simulink model "PH1_2converters_psv"  (R2017a)
settings: Solver=VariableStepAuto  StartTime=0.0  StopTime=.2  MaxStep=1e-4  RelTol=1e-3
libraries: powerlib x35, powerlib_meascontrol x2
settings Model: Creator=erich  LastModifiedBy=erich

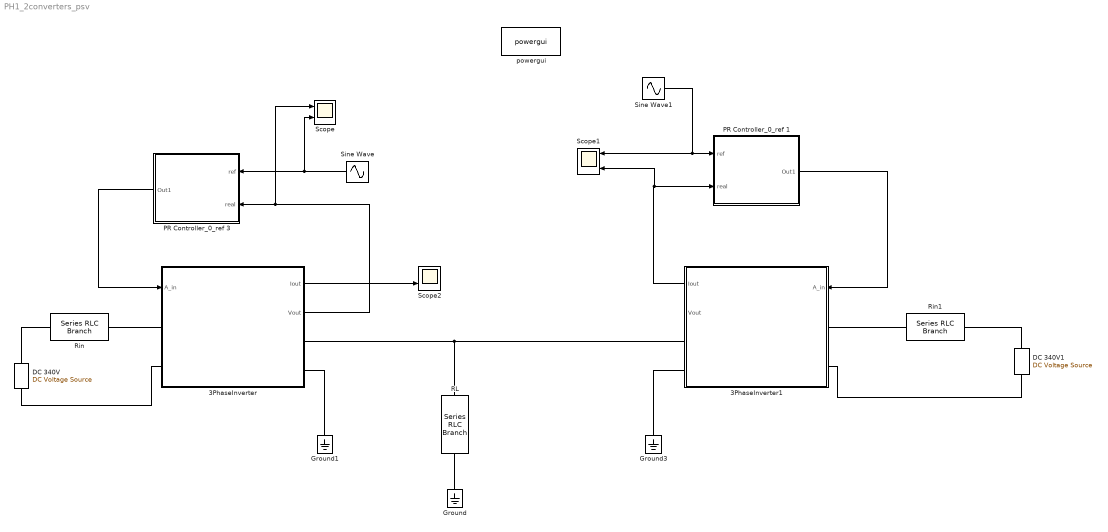
== system PH1_2converters_psv ==
  3PhaseInverter : Subsystem  mask{st_time=2e-3, f_sw=5000}
      mask prompts: st_time "Tiempo muerto (Start)"; f_sw "Switching frequency"
      mask Display:
      | port_label('input', 1, 'd', 'texmode', 'on')
      | 
      | port_label('lconn', 1, 'DC +')
      | port_label('lconn', 2, 'DC -')
      | 
      | 
      | port_label('rconn', 1, 'V_{out+}')
      | port_label('rconn', 2, 'B_{out-}')
      | 
      | 
      | port_label('output', 1, 'I_{out}', 'texmode', 'on')
      | port_label('output', 2, 'V_{out}', 'texmode', 'on')
      | 
      | plot([0.1 .9], [0.1 .9])
      | plot([0.2 .4], [.7 .7])
      | plot([0.2 .24], [.65 .65])
      | plot([0.28 .32], [.65 .65])
      | plot([0.36 .40], [.65 .65])
      | 
      | plot([.5:.01:.7], .25+sin(30*[.2:.01:.4])/10)
  3PhaseInverter1 : Subsystem  mask{st_time=.1, f_sw=5000}
      mask prompts: st_time "Tiempo muerto (Start)"; f_sw "Switching frequency"
      mask Display:
      | port_label('input', 1, 'd', 'texmode', 'on')
      | 
      | port_label('lconn', 1, 'DC +')
      | port_label('lconn', 2, 'DC -')
      | 
      | 
      | port_label('rconn', 1, 'V_{out+}')
      | port_label('rconn', 2, 'B_{out-}')
      | 
      | 
      | port_label('output', 1, 'I_{out}', 'texmode', 'on')
      | port_label('output', 2, 'V_{out}', 'texmode', 'on')
      | 
      | plot([0.1 .9], [0.1 .9])
      | plot([0.2 .4], [.7 .7])
      | plot([0.2 .24], [.65 .65])
      | plot([0.28 .32], [.65 .65])
      | plot([0.36 .40], [.65 .65])
      | 
      | plot([.5:.01:.7], .25+sin(30*[.2:.01:.4])/10)
  DC 340V : powerlib/Electrical Sources/DC Voltage Source  Amplitude=340  Measurements=None
  DC 340V1 : powerlib/Electrical Sources/DC Voltage Source  Amplitude=340  Measurements=None
  Ground : powerlib/Elements/Ground  LConnTagsString=a
  Ground1 : powerlib/Elements/Ground  LConnTagsString=a
  Ground3 : powerlib/Elements/Ground  LConnTagsString=a
  PR Controller_0_ref 1 : Subsystem  mask{Kp=1/100, Ki=7, wa=10, w0=60*2*pi, st_time=.1}
      mask prompts: Kp "Ganancia Proporcional"; Ki "Ganancia Integral"; wa "Ancho camapana resonancia"; w0 "Frecuencia Central"; st_time "Tiempo muerto (Start)"
      mask Display:
      | port_label('input',1,'ref')
      | port_label('input',2,'sens')
      | port_label('output',1,'out')
      | 
      | plot(.4+[0:.01:pi/10], .32+sin(40*[0:.01:pi/10])/13)
      | 
      | plot([.4 .6],.05+[.5 .7])
      | plot([.4 .6],.05+[.9 .7])
      | plot([.4 .4],.05+[.9 .5])
      | 
      | text(.27,.37,'\fontsize{25} \int', 'texmode', 'on')
  PR Controller_0_ref 3 : Subsystem  mask{Kp=1/100, Ki=1, wa=1, w0=60*2*pi, st_time=2e-3}
      mask prompts: Kp "Ganancia Proporcional"; Ki "Ganancia Integral"; wa "Ancho camapana resonancia"; w0 "Frecuencia Central"; st_time "Tiempo muerto (Start)"
      mask Display:
      | port_label('input',1,'ref')
      | port_label('input',2,'sens')
      | port_label('output',1,'out')
      | 
      | plot(.4+[0:.01:pi/10], .32+sin(40*[0:.01:pi/10])/13)
      | 
      | plot([.4 .6],.05+[.5 .7])
      | plot([.4 .6],.05+[.9 .7])
      | plot([.4 .4],.05+[.9 .5])
      | 
      | text(.27,.37,'\fontsize{25} \int', 'texmode', 'on')
  RL : powerlib/Elements/Series RLC Branch  LConnTagsString=__new0  RConnTagsString=__new0  BranchType=R  Resistance=30  Inductance=500e-3  SetiL0=off  InitialCurrent=0  Capacitance=100e-6  Setx0=off  InitialVoltage=0  Measurements=None
  Rin : powerlib/Elements/Series RLC Branch  LConnTagsString=__new0  RConnTagsString=__new0  BranchType=R  Resistance=.01  Inductance=0  SetiL0=off  InitialCurrent=0  Capacitance=0  Setx0=off  InitialVoltage=0  Measurements=None
  Rin1 : powerlib/Elements/Series RLC Branch  LConnTagsString=__new0  RConnTagsString=__new0  BranchType=R  Resistance=.01  Inductance=0  SetiL0=off  InitialCurrent=0  Capacitance=0  Setx0=off  InitialVoltage=0  Measurements=None
  Scope : Scope  NumInputPorts=2
  Scope1 : Scope  NumInputPorts=2
  Scope2 : Scope  NumInputPorts=2
  Sine Wave : Sin  Amplitude=170  Frequency=2*pi*60  SampleTime=0
  Sine Wave1 : Sin  Amplitude=3  Frequency=2*pi*60  SampleTime=0
  powergui : powerlib/powergui  Priority=1  SimulationMode=Continuous  SampleTime=50e-6  frequency=60  Iterations=50  frequencyindice=0  Pbase=100e6  ErrMax=1e-4  UnitsV=kV  UnitsW=MW  buscounter=0  FunctionMessages=off  echomessages=off  EnableUseOfTLC=off  CurrentSourceSwitches=off  DisableSnubberDevices=off  DisableRonSwitches=off  DisableVfSwitches=off  DisplayEquations=off  SolverType=Tustin/Backward Euler (TBE)  Interpol=off  ExternalGateDelay=off  methode=off  Ts=100  x0status=blocks  SPID=on  SwTol=0  HookPort=off  RestoreLinks=warning  ResistiveCurrentMeasurement=off  Frange=[0:2:500]  Ylog=off  Xlog=on  ShowGrid=off  save=off  variable=ZData  structure=0  ZoomFFT=off  StartTime=0.0  cycles=1  DisplayStyle=1  fundamental=60  FreqAxis=off  MaxFrequency=1000  frequencyindicesteady=1  RmsSteady=1  display=off
  wires:
  3PhaseInverter/2(Vout) -> Scope/1, PR Controller_0_ref 3/2(real)
  Sine Wave/1 -> Scope/2, PR Controller_0_ref 3/1(ref)
  PR Controller_0_ref 3/1(Out1) -> 3PhaseInverter/1(A_in)
  Sine Wave1/1 -> PR Controller_0_ref 1/1(ref), Scope1/1
  3PhaseInverter1/1(Iout) -> Scope1/2, PR Controller_0_ref 1/2(real)
  PR Controller_0_ref 1/1(Out1) -> 3PhaseInverter1/1(A_in)
  3PhaseInverter/1(Iout) -> Scope2/2
  connections:
  RL/LConn1 -- 3PhaseInverter/RConn1 -- 3PhaseInverter1/RConn1
  Ground/LConn1 -- RL/RConn1
  3PhaseInverter/RConn2 -- Ground1/LConn1
  DC 340V/LConn1 -- 3PhaseInverter/LConn2
  DC 340V/RConn1 -- Rin/LConn1
  Rin/RConn1 -- 3PhaseInverter/LConn1
  DC 340V1/RConn1 -- Rin1/LConn1
  3PhaseInverter1/RConn2 -- Ground3/LConn1
  DC 340V1/LConn1 -- 3PhaseInverter1/LConn2
  Rin1/RConn1 -- 3PhaseInverter1/LConn1

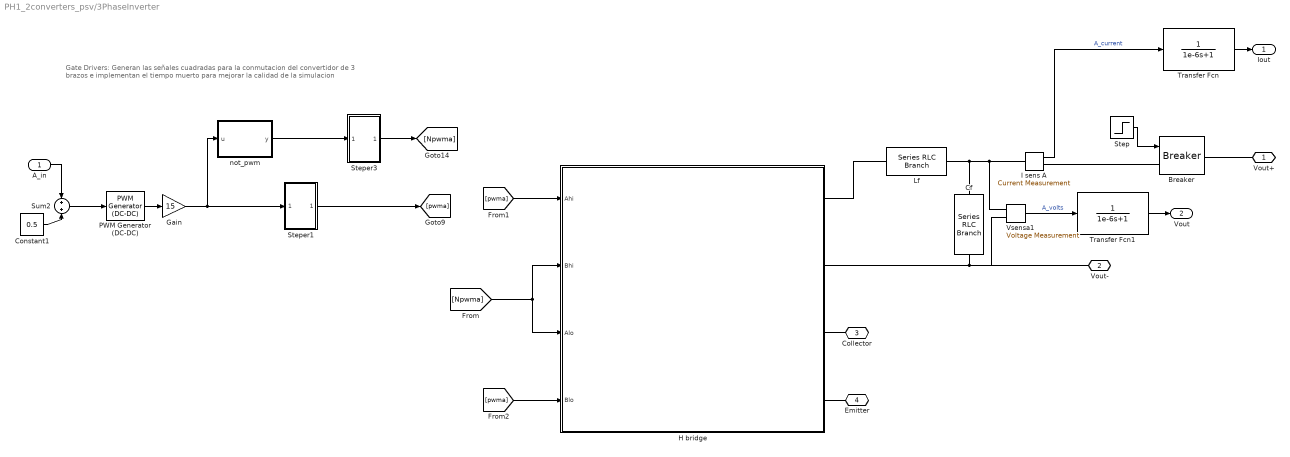
== system PH1_2converters_psv/3PhaseInverter ==
  note: Gate Drivers: Generan las señales cuadradas para
      | la conmutacion del convertidor de 3 brazos e implementan el
      | tiempo muerto para mejorar la calidad de la simulacion
  A_in : Inport
  Breaker : powerlib/Elements/Breaker  InitialState=0  SwitchingTimes="[1/60  5/60]"  External=on  BreakerResistance=0.01  SnubberResistance=1e6  SnubberCapacitance=inf  Measurements=None  MoreParameters=on  NoBreakLoop=off
      settings: SourceProductName=Simscape Power Systems
  Cf : powerlib/Elements/Series RLC Branch  LConnTagsString=__new0  RConnTagsString=__new0  BranchType=C  Resistance=1  Inductance=1e-3  SetiL0=off  InitialCurrent=0  Capacitance=2.2e-6  Setx0=off  InitialVoltage=0  Measurements=None
  Constant1 : Constant  Value=0.5
  Gain : Gain  Gain=15
  H bridge : Subsystem
      mask Display:
      | port_label('input', 1, '\fontsize{12} Ahi', 'texmode', 'on')
      | port_label('input', 2, '\fontsize{12} Alo', 'texmode', 'on')
      | port_label('input', 3, '\fontsize{12} Bhi', 'texmode', 'on')
      | port_label('input', 4, '\fontsize{12} Blo', 'texmode', 'on')
      | 
      | 
      | port_label('rconn', 1, '\fontsize{12} V_{out} +', 'texmode', 'on')
      | port_label('rconn', 2, '\fontsize{12} V_{out} -', 'texmode', 'on')
      | 
      | port_label('rconn', 3, '\fontsize{12} Collector', 'texmode', 'on')
      | port_label('rconn', 4, '\fontsize{12} Emitter', 'texmode', 'on')
      | 
      | lvx = [.1 .1];
      | lvy = [.1 .2];
      | lhx = [.1 .2];
      | lhy = [.1 .1];
      | 
      | 
      | % se dibujan los interruptores de la izquierda
      | plot(lvx+.07, lvy*.8+.028+.1)
      | plot(lvx+.1, lvy+.1)
      | plot(lhx*.5+.15, lhy+.1)
      | plot(lhx*.5+.15, lhy+.2)
      | plot(lhx*.5+.07, lhy+.15)
      | 
      | d=0.5;
      | 
      | plot(lvx+.07, lvy*.8+.028+.1+d)
      | plot(lvx+.1, lvy+.1+d)
      | plot(lhx*.5+.15, lhy+.1+d)
      | plot(lhx*.5+.15, lhy+.2+d)
      | plot(lhx*.5+.07, lhy+.15+d)
      | 
      | 
      | % se dibujan los interruptores del medio
      | h=.3;
      | 
      | %plot(lvx+.07+h, lvy*.8+.028+.1)
      | %plot(lvx+.1+h, lvy+.1)
      | %plot(lhx*.5+.15+h, lhy+.1)
      | %plot(lhx*.5+.15+h, lhy+.2)
      | %plot(lhx*.5+.07+h, lhy+.15)
      | 
      | %plot(lvx+.07+h, lvy*.8+.028+.1+d)
      | %plot(lvx+.1+h, lvy+.1+d)
      | %plot(lhx*.5+.15+h, lhy+.1+d)
      | %plot(lhx*.5+.15+h, lhy+.2+d)
      | %plot(lhx*.5+.07+h, lhy+.15+d)
      | 
      | % se dibujan los interruptores de la derecha
      | h=.6
      | 
      | plot(lvx+.07+h, lvy*.8+.028+.1)
      | plot(lvx+.1+h, lvy+.1)
      | plot(lhx*.5+.15+h, lhy+.1)
      | plot(lhx*.5+.15+h, lhy+.2)
      | plot(lhx*.5+.07+h, lhy+.15)
      | 
      | plot(lvx+.07+h, lvy*.8+.028+.1+d)
      | plot(lvx+.1+h, lvy+.1+d)
      | plot(lhx*.5+.15+h, lhy+.1+d)
      | plot(lhx*.5+.15+h, lhy+.2+d)
      | plot(lhx*.5+.07+h, lhy+.15+d)
      | 
      | 
      | % se conectan los interruptores.
      | plot(lvx+.15, lvy*4-.1)
      | %plot(lvx+.15+.3, lvy*4-.1)
      | plot(lvx+.15+.6, lvy*4-.1)
      | 
      | 
      | plot(lvx+.15, lvy+.7)
      | %plot(lvx+.15+.3, lvy+.7)
      | plot(lvx+.15+.6, lvy+.7)
      | 
      | plot(lvx+.15, lvy)
      | %plot(lvx+.15+.3, lvy)
      | plot(lvx+.15+.6, lvy)
      | 
      | plot(lhx*6-.35, lhy)
      | plot(lhx*6-.35, lhy+.8)
      | 
      | % raul esteban alzate 313 515 86 11
  I sens A : powerlib/Measurements/Current Measurement  PhasorSimulation=off  OutputType=Complex  PSBequivalent=0
  Lf : powerlib/Elements/Series RLC Branch  LConnTagsString=__new0  RConnTagsString=__new0  BranchType=RL  Resistance=.1  Inductance=10e-3  SetiL0=off  InitialCurrent=0  Capacitance=1e-6  Setx0=off  InitialVoltage=0  Measurements=None
  PWM Generator (DC-DC) : powerlib_meascontrol/Pulse & Signal Generators/PWM Generator (DC-DC)  Fsw=f_sw  Ts=0
  Step : Step  Time=st_time  SampleTime=0
  Steper1 : Subsystem
  Steper3 : Subsystem
  Sum2 : Sum
  Transfer Fcn : TransferFcn  Denominator=[1e-6 1]
  Transfer Fcn1 : TransferFcn  Denominator=[1e-6 1]
  Vsensa1 : powerlib/Measurements/Voltage Measurement  PhasorSimulation=off  OutputType=Complex  PSBequivalent=0
  not_pwm : MATLAB Function  TreatAsAtomicUnit=on
  Vout+ : PMIOPort  Port=1  Side=Right
  Vout- : PMIOPort  Port=2  Side=Right
  Collector : PMIOPort  Port=3  Side=Left
  Emitter : PMIOPort  Port=4  Side=Left
  Iout : Outport
  Vout : Outport  Port=2
  wires:
  not_pwm/1(y) -> Steper3/1(In1)
  Sum2/1 -> PWM Generator (DC-DC)/1
  PWM Generator (DC-DC)/1 -> Gain/1
  Constant1/1 -> Sum2/2
  A_in/1 -> Sum2/1
  Steper1/1(Out1) -> [pwma]
  Steper3/1(Out1) -> [Npwma]
  Gain/1 -> Steper1/1(In1), not_pwm/1(u)
  [pwma] -> H bridge/1(Ahi)
  [Npwma] -> H bridge/2(Bhi), H bridge/3(Alo)
  [pwma] -> H bridge/4(Blo)
  I sens A/1 -> Transfer Fcn/1  "A_current"
  Vsensa1/1 -> Transfer Fcn1/1  "A_volts"
  Transfer Fcn/1 -> Iout/1
  Transfer Fcn1/1 -> Vout/1
  Step/1 -> Breaker/1
  connections:
  H bridge/RConn3 -- Collector/RConn1
  H bridge/RConn4 -- Emitter/RConn1
  Lf/LConn1 -- H bridge/RConn1
  I sens A/LConn1 -- Cf/LConn1 -- Lf/RConn1 -- Vsensa1/LConn1
  H bridge/RConn2 -- Vout-/RConn1 -- Vsensa1/LConn2 -- Cf/RConn1
  Breaker/LConn1 -- I sens A/RConn1
  Breaker/RConn1 -- Vout+/RConn1

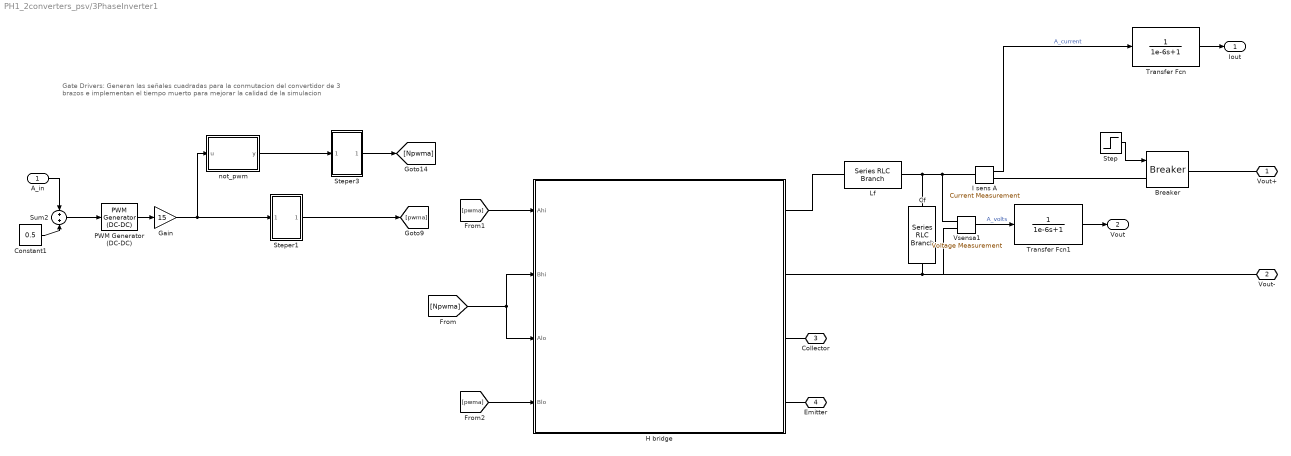
== system PH1_2converters_psv/3PhaseInverter1 ==
  note: Gate Drivers: Generan las señales cuadradas para
      | la conmutacion del convertidor de 3 brazos e implementan el
      | tiempo muerto para mejorar la calidad de la simulacion
  A_in : Inport
  Breaker : powerlib/Elements/Breaker  InitialState=0  SwitchingTimes="[1/60  5/60]"  External=on  BreakerResistance=0.01  SnubberResistance=1e6  SnubberCapacitance=inf  Measurements=None  MoreParameters=on  NoBreakLoop=off
      settings: SourceProductName=Simscape Power Systems
  Cf : powerlib/Elements/Series RLC Branch  LConnTagsString=__new0  RConnTagsString=__new0  BranchType=C  Resistance=1  Inductance=1e-3  SetiL0=off  InitialCurrent=0  Capacitance=2.2e-6  Setx0=off  InitialVoltage=0  Measurements=None
  Constant1 : Constant  Value=0.5
  Gain : Gain  Gain=15
  H bridge : Subsystem
      mask Display:
      | port_label('input', 1, '\fontsize{12} Ahi', 'texmode', 'on')
      | port_label('input', 2, '\fontsize{12} Alo', 'texmode', 'on')
      | port_label('input', 3, '\fontsize{12} Bhi', 'texmode', 'on')
      | port_label('input', 4, '\fontsize{12} Blo', 'texmode', 'on')
      | 
      | 
      | port_label('rconn', 1, '\fontsize{12} V_{out} +', 'texmode', 'on')
      | port_label('rconn', 2, '\fontsize{12} V_{out} -', 'texmode', 'on')
      | 
      | port_label('rconn', 3, '\fontsize{12} Collector', 'texmode', 'on')
      | port_label('rconn', 4, '\fontsize{12} Emitter', 'texmode', 'on')
      | 
      | lvx = [.1 .1];
      | lvy = [.1 .2];
      | lhx = [.1 .2];
      | lhy = [.1 .1];
      | 
      | 
      | % se dibujan los interruptores de la izquierda
      | plot(lvx+.07, lvy*.8+.028+.1)
      | plot(lvx+.1, lvy+.1)
      | plot(lhx*.5+.15, lhy+.1)
      | plot(lhx*.5+.15, lhy+.2)
      | plot(lhx*.5+.07, lhy+.15)
      | 
      | d=0.5;
      | 
      | plot(lvx+.07, lvy*.8+.028+.1+d)
      | plot(lvx+.1, lvy+.1+d)
      | plot(lhx*.5+.15, lhy+.1+d)
      | plot(lhx*.5+.15, lhy+.2+d)
      | plot(lhx*.5+.07, lhy+.15+d)
      | 
      | 
      | % se dibujan los interruptores del medio
      | h=.3;
      | 
      | %plot(lvx+.07+h, lvy*.8+.028+.1)
      | %plot(lvx+.1+h, lvy+.1)
      | %plot(lhx*.5+.15+h, lhy+.1)
      | %plot(lhx*.5+.15+h, lhy+.2)
      | %plot(lhx*.5+.07+h, lhy+.15)
      | 
      | %plot(lvx+.07+h, lvy*.8+.028+.1+d)
      | %plot(lvx+.1+h, lvy+.1+d)
      | %plot(lhx*.5+.15+h, lhy+.1+d)
      | %plot(lhx*.5+.15+h, lhy+.2+d)
      | %plot(lhx*.5+.07+h, lhy+.15+d)
      | 
      | % se dibujan los interruptores de la derecha
      | h=.6
      | 
      | plot(lvx+.07+h, lvy*.8+.028+.1)
      | plot(lvx+.1+h, lvy+.1)
      | plot(lhx*.5+.15+h, lhy+.1)
      | plot(lhx*.5+.15+h, lhy+.2)
      | plot(lhx*.5+.07+h, lhy+.15)
      | 
      | plot(lvx+.07+h, lvy*.8+.028+.1+d)
      | plot(lvx+.1+h, lvy+.1+d)
      | plot(lhx*.5+.15+h, lhy+.1+d)
      | plot(lhx*.5+.15+h, lhy+.2+d)
      | plot(lhx*.5+.07+h, lhy+.15+d)
      | 
      | 
      | % se conectan los interruptores.
      | plot(lvx+.15, lvy*4-.1)
      | %plot(lvx+.15+.3, lvy*4-.1)
      | plot(lvx+.15+.6, lvy*4-.1)
      | 
      | 
      | plot(lvx+.15, lvy+.7)
      | %plot(lvx+.15+.3, lvy+.7)
      | plot(lvx+.15+.6, lvy+.7)
      | 
      | plot(lvx+.15, lvy)
      | %plot(lvx+.15+.3, lvy)
      | plot(lvx+.15+.6, lvy)
      | 
      | plot(lhx*6-.35, lhy)
      | plot(lhx*6-.35, lhy+.8)
      | 
      | % raul esteban alzate 313 515 86 11
  I sens A : powerlib/Measurements/Current Measurement  PhasorSimulation=off  OutputType=Complex  PSBequivalent=0
  Lf : powerlib/Elements/Series RLC Branch  LConnTagsString=__new0  RConnTagsString=__new0  BranchType=RL  Resistance=.1  Inductance=10e-3  SetiL0=off  InitialCurrent=0  Capacitance=1e-6  Setx0=off  InitialVoltage=0  Measurements=None
  PWM Generator (DC-DC) : powerlib_meascontrol/Pulse & Signal Generators/PWM Generator (DC-DC)  Fsw=f_sw  Ts=0
  Step : Step  Time=st_time  SampleTime=0
  Steper1 : Subsystem
  Steper3 : Subsystem
  Sum2 : Sum
  Transfer Fcn : TransferFcn  Denominator=[1e-6 1]
  Transfer Fcn1 : TransferFcn  Denominator=[1e-6 1]
  Vsensa1 : powerlib/Measurements/Voltage Measurement  PhasorSimulation=off  OutputType=Complex  PSBequivalent=0
  not_pwm : MATLAB Function  TreatAsAtomicUnit=on
  Vout+ : PMIOPort  Port=1  Side=Right
  Vout- : PMIOPort  Port=2  Side=Right
  Collector : PMIOPort  Port=3  Side=Left
  Emitter : PMIOPort  Port=4  Side=Left
  Iout : Outport
  Vout : Outport  Port=2
  wires:
  Vsensa1/1 -> Transfer Fcn1/1  "A_volts"
  I sens A/1 -> Transfer Fcn/1  "A_current"
  [pwma] -> H bridge/4(Blo)
  [Npwma] -> H bridge/3(Alo), H bridge/2(Bhi)
  [pwma] -> H bridge/1(Ahi)
  Gain/1 -> not_pwm/1(u), Steper1/1(In1)
  Steper3/1(Out1) -> [Npwma]
  Steper1/1(Out1) -> [pwma]
  A_in/1 -> Sum2/1
  Constant1/1 -> Sum2/2
  PWM Generator (DC-DC)/1 -> Gain/1
  Sum2/1 -> PWM Generator (DC-DC)/1
  not_pwm/1(y) -> Steper3/1(In1)
  Transfer Fcn/1 -> Iout/1
  Transfer Fcn1/1 -> Vout/1
  Step/1 -> Breaker/1
  connections:
  Cf/RConn1 -- Vsensa1/LConn2 -- Vout-/RConn1 -- H bridge/RConn2
  Vsensa1/LConn1 -- Lf/RConn1 -- Cf/LConn1 -- I sens A/LConn1
  Lf/LConn1 -- H bridge/RConn1
  H bridge/RConn4 -- Emitter/RConn1
  H bridge/RConn3 -- Collector/RConn1
  Breaker/LConn1 -- I sens A/RConn1
  Breaker/RConn1 -- Vout+/RConn1

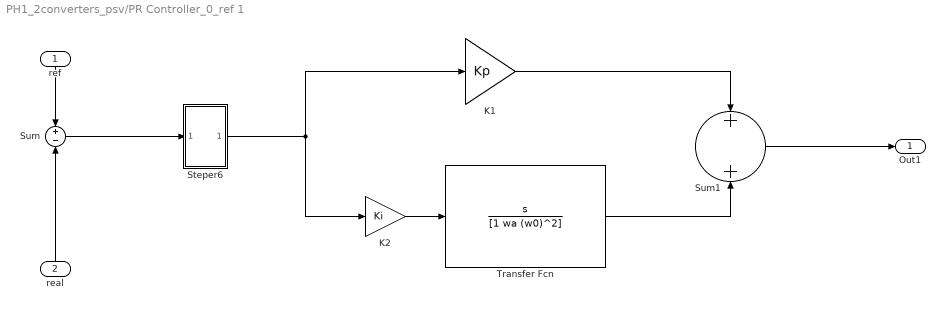
== system PH1_2converters_psv/PR Controller_0_ref 1 ==
  ref : Inport
  real : Inport  Port=2
  K1 : Gain  Gain=Kp
  K2 : Gain  Gain=Ki
  Steper6 : Subsystem
  Sum : Sum  Inputs=+-
  Sum1 : Sum  Inputs=+|+
  Transfer Fcn : TransferFcn  Numerator=[1 0]  Denominator=[1 wa (w0)^2]
  Out1 : Outport
  wires:
  Sum1/1 -> Out1/1
  Steper6/1(Out1) -> K2/1, K1/1
  K2/1 -> Transfer Fcn/1
  Transfer Fcn/1 -> Sum1/2
  K1/1 -> Sum1/1
  Sum/1 -> Steper6/1(In1)
  ref/1 -> Sum/1
  real/1 -> Sum/2

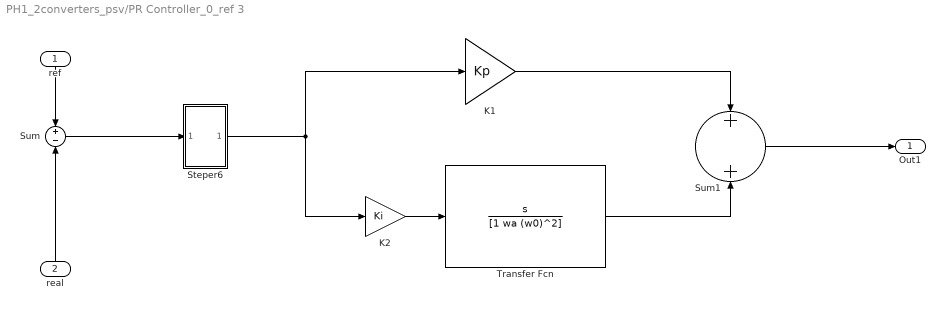
== system PH1_2converters_psv/PR Controller_0_ref 3 ==
  ref : Inport
  real : Inport  Port=2
  K1 : Gain  Gain=Kp
  K2 : Gain  Gain=Ki
  Steper6 : Subsystem
  Sum : Sum  Inputs=+-
  Sum1 : Sum  Inputs=+|+
  Transfer Fcn : TransferFcn  Numerator=[1 0]  Denominator=[1 wa (w0)^2]
  Out1 : Outport
  wires:
  real/1 -> Sum/2
  ref/1 -> Sum/1
  Sum/1 -> Steper6/1(In1)
  K1/1 -> Sum1/1
  Transfer Fcn/1 -> Sum1/2
  K2/1 -> Transfer Fcn/1
  Steper6/1(Out1) -> K1/1, K2/1
  Sum1/1 -> Out1/1

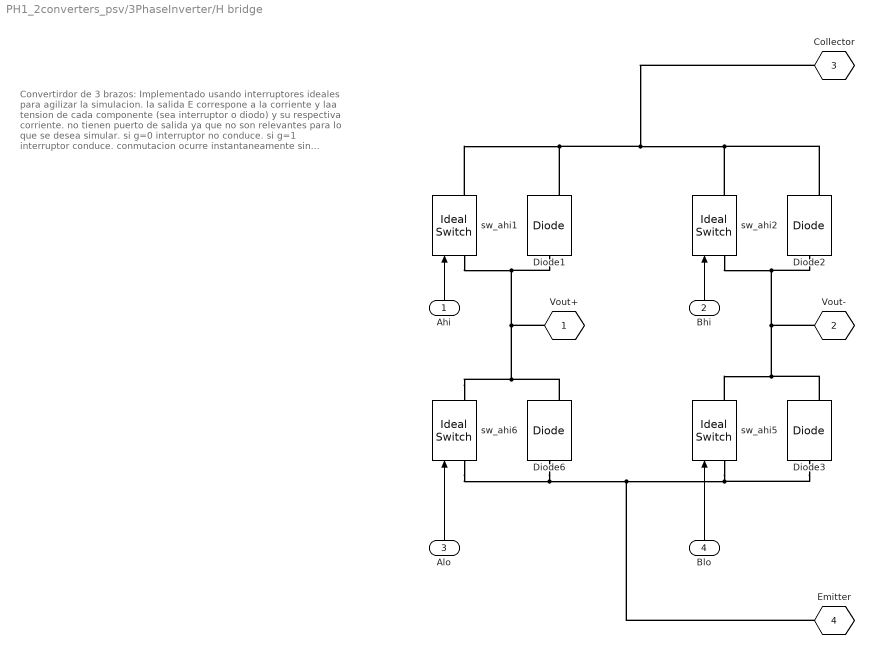
== system PH1_2converters_psv/3PhaseInverter/H bridge ==
  note: Convertirdor de 3 brazos:
      |
      | Implementado usando interruptores
      | ideales para agilizar la simulacion.
      | la salida E correspone a la corriente y laa
      | tension de cada componente
      | (sea interruptor o diodo) y su respectiva
      | corriente. no tienen puerto de salida ya que no
      | son relevantes para lo que se desea simular.
      |
      | si g=0 interruptor no conduce.
      | si g=1 interruptor conduce.
      |
      | conmutacion ocurre instantaneamente sin
      | retardo.
  Ahi : Inport
  Bhi : Inport  Port=2
  Alo : Inport  Port=3
  Blo : Inport  Port=4
   sw_ahi{1..2,5..6} (4 alike) : powerlib/Power Electronics/Ideal Switch  Ron=0.1  Lon=0  IC=0  Rs=1e6  Cs=10e-12  Measurements=on
  Diode{1..3,6} (4 alike) : powerlib/Power Electronics/Diode  Ron=.2  Lon=0  Vf=0.8  IC=0  UseSnubber=0  Rs=0  Cs=0  Measurements=on
  " Vout+" : PMIOPort  Tag=PMCPort  Port=1  Side=Right
  Vout- : PMIOPort  Tag=PMCPort  Port=2  Side=Right
  Collector : PMIOPort  Tag=PMCPort  Port=3  Side=Right
  Emitter : PMIOPort  Tag=PMCPort  Port=4  Side=Right
  wires:
  Alo/1 -> " sw_ahi6"/1
  Ahi/1 -> " sw_ahi1"/1
  Blo/1 -> " sw_ahi5"/1
  Bhi/1 -> " sw_ahi2"/1
  connections:
  Diode3/RConn1 -- Vout-/RConn1 -- " sw_ahi2"/LConn1 -- Diode2/LConn1 -- " sw_ahi5"/RConn1
  Diode3/LConn1 -- Emitter/RConn1 -- Diode6/LConn1 -- " sw_ahi6"/LConn1 -- " sw_ahi5"/LConn1
  Diode2/RConn1 -- Collector/RConn1 -- " sw_ahi1"/RConn1 -- Diode1/RConn1 -- " sw_ahi2"/RConn1
  " sw_ahi6"/RConn1 -- Diode6/RConn1 -- " Vout+"/RConn1 -- Diode1/LConn1 -- " sw_ahi1"/LConn1

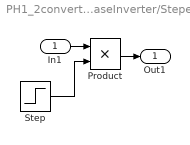
== system PH1_2converters_psv/3PhaseInverter/Steper1 ==
  In1 : Inport
  Product : Product
  Step : Step  Time=st_time  SampleTime=0
  Out1 : Outport
  wires:
  Step/1 -> Product/2
  In1/1 -> Product/1
  Product/1 -> Out1/1

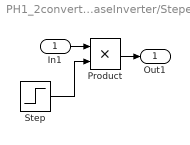
== system PH1_2converters_psv/3PhaseInverter/Steper3 ==
  In1 : Inport
  Product : Product
  Step : Step  Time=st_time  SampleTime=0
  Out1 : Outport
  wires:
  Product/1 -> Out1/1
  In1/1 -> Product/1
  Step/1 -> Product/2

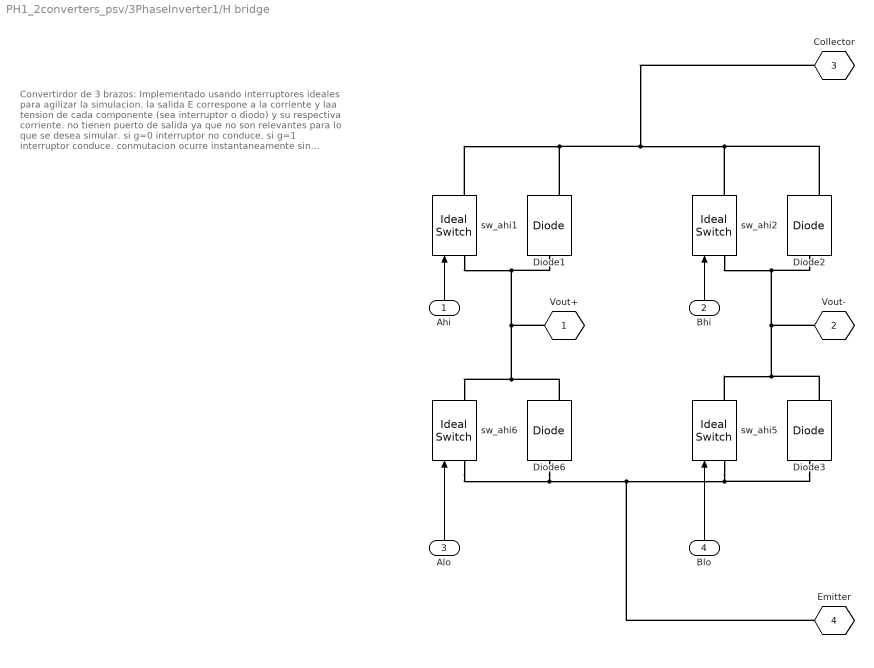
== system PH1_2converters_psv/3PhaseInverter1/H bridge ==
  note: Convertirdor de 3 brazos:
      |
      | Implementado usando interruptores
      | ideales para agilizar la simulacion.
      | la salida E correspone a la corriente y laa
      | tension de cada componente
      | (sea interruptor o diodo) y su respectiva
      | corriente. no tienen puerto de salida ya que no
      | son relevantes para lo que se desea simular.
      |
      | si g=0 interruptor no conduce.
      | si g=1 interruptor conduce.
      |
      | conmutacion ocurre instantaneamente sin
      | retardo.
  Ahi : Inport
  Bhi : Inport  Port=2
  Alo : Inport  Port=3
  Blo : Inport  Port=4
   sw_ahi{1..2,5..6} (4 alike) : powerlib/Power Electronics/Ideal Switch  Ron=0.1  Lon=0  IC=0  Rs=1e6  Cs=10e-12  Measurements=on
  Diode{1..3,6} (4 alike) : powerlib/Power Electronics/Diode  Ron=.2  Lon=0  Vf=0.8  IC=0  UseSnubber=0  Rs=0  Cs=0  Measurements=on
  " Vout+" : PMIOPort  Tag=PMCPort  Port=1  Side=Right
  Vout- : PMIOPort  Tag=PMCPort  Port=2  Side=Right
  Collector : PMIOPort  Tag=PMCPort  Port=3  Side=Right
  Emitter : PMIOPort  Tag=PMCPort  Port=4  Side=Right
  wires:
  Bhi/1 -> " sw_ahi2"/1
  Blo/1 -> " sw_ahi5"/1
  Ahi/1 -> " sw_ahi1"/1
  Alo/1 -> " sw_ahi6"/1
  connections:
  " sw_ahi1"/LConn1 -- Diode1/LConn1 -- " Vout+"/RConn1 -- Diode6/RConn1 -- " sw_ahi6"/RConn1
  " sw_ahi2"/RConn1 -- Diode1/RConn1 -- " sw_ahi1"/RConn1 -- Collector/RConn1 -- Diode2/RConn1
  " sw_ahi5"/LConn1 -- " sw_ahi6"/LConn1 -- Diode6/LConn1 -- Emitter/RConn1 -- Diode3/LConn1
  " sw_ahi5"/RConn1 -- Diode2/LConn1 -- " sw_ahi2"/LConn1 -- Vout-/RConn1 -- Diode3/RConn1

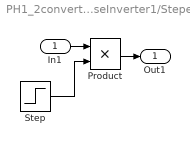
== system PH1_2converters_psv/3PhaseInverter1/Steper1 ==
  In1 : Inport
  Product : Product
  Step : Step  Time=st_time  SampleTime=0
  Out1 : Outport
  wires:
  Product/1 -> Out1/1
  In1/1 -> Product/1
  Step/1 -> Product/2

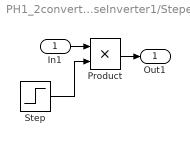
== system PH1_2converters_psv/3PhaseInverter1/Steper3 ==
  In1 : Inport
  Product : Product
  Step : Step  Time=st_time  SampleTime=0
  Out1 : Outport
  wires:
  Step/1 -> Product/2
  In1/1 -> Product/1
  Product/1 -> Out1/1

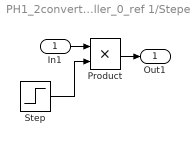
== system PH1_2converters_psv/PR Controller_0_ref 1/Steper6 ==
  In1 : Inport
  Product : Product
  Step : Step  Time=st_time  SampleTime=0
  Out1 : Outport
  wires:
  Step/1 -> Product/2
  In1/1 -> Product/1
  Product/1 -> Out1/1

== system PH1_2converters_psv/PR Controller_0_ref 3/Steper6 ==
  In1 : Inport
  Product : Product
  Step : Step  Time=st_time  SampleTime=0
  Out1 : Outport
  wires:
  Product/1 -> Out1/1
  In1/1 -> Product/1
  Step/1 -> Product/2

== matlab function PH1_2converters_psv/3PhaseInverter1/not_pwm ==
  data: u input; y output
function y = fcn(u)
%#codegen

if(u==0 || u<0)
    a=15;
else
    a=0;
end;

y = a;

== matlab function PH1_2converters_psv/3PhaseInverter/not_pwm ==
  data: u input; y output
function y = fcn(u)
%#codegen

if(u==0 || u<0)
    a=15;
else
    a=0;
end;

y = a;
